simulink model "KUKA_EE_Controller_v22_orbital_verification2"  (R2024a)
settings: Solver=VariableStepAuto  StartTime=0.0  StopTime=120  FixedStep=0.01  RelTol=1e-3
InitFcn:
  | %rho_0t=[0.29;0.29;0.29]; %m
  | %V_0t=[-0.001;-0.001;0];%[-0.0005;-0.0005;0];
  | %w_t=[0;0;-0.002];
  | 
  | 
  | %rho_0t=[0.3;0.3;0.2]; %m
  | %V_0t=[-0.001;-0.001;0];%[-0.0005;-0.0005;0];
  | %w_t=[0;0;-0.001];
values from neighbouring files (symbols this model uses):
  e_orbit = 0    [Initiate_FQ.m]
  e_orbit_t = (mu_orbit_t^2/mu_earth)/radius_orbit_t-1    [Initiate_FQ.m]
  g_cm = zeros(4,4,n)    [Initiate_KUKA_inv.m]    (also in KUKA_Main.m)
  M0 = M_temp.M0.data(:,:,1)    [Initiate_FQ.m]    (also in KUKA_Main.m)
  m0 = robot.Bodies{1,n+1}.Mass    [Initiate_KUKA_inv.m]    (also in KUKA_Main.m)
  m0_frak = diag_M(1:6,1:6)    [Initiate_KUKA_inv.m]
  M0m = M_temp.M0m.data(:,:,1)    [Initiate_FQ.m]    (also in KUKA_Main.m)
  m_diag = diag_M(7:end,7:end)    [Initiate_KUKA_inv.m]
  Mean_Anomaly0 = MeanAnomaly(e_orbit,E0)    [Initiate_FQ.m]
  Mean_Anomaly0_t = MeanAnomaly(e_orbit,E0)    [Initiate_FQ.m]
  Mm = simplify(transpose(Xi_m)*transpose(Lm)*diagM*Lm*Xi_m)    [KUKA_Main.m]
  mm = zeros(1,n)    [Initiate_KUKA_inv.m]    (also in KUKA_Main.m)
  mu = P0    [Initiate_FQ.m]    (also in Initiate_KUKA_inv.m = zeros(6,1); KUKA_Main.m = P)
  mu_earth = 3.986004418*10^14    (= 398600441800000)    [Initiate_FQ.m]
  mu_orbit = sqrt(radius_orbit*mu_earth)    [Initiate_FQ.m]
  mu_orbit_t = radius_orbit_t*vel_orbit_t    [Initiate_FQ.m]
  n_orbit = (mu_earth^2)/(mu_orbit^3)    [Initiate_FQ.m]
  n_orbit_t = (mu_earth^2)/(mu_orbit^3)    [Initiate_FQ.m]
  q_dot_m = [0;0;0;0;0;0;0]    [Initiate_FQ.m]    (also in Initiate_KUKA_inv.m; KUKA_Main.m = [qdot1;qdot2;qdot3;qdot4;qdot5;qdot6;qdot7])
  q_m = [0.2;1.2;0.3;2.5;0.5;1.5;0.6]    [Initiate_FQ.m]    (also in Initiate_KUKA_inv.m = [0;0;0;0;0;0;0]; KUKA_Main.m = [q_m1;q_m2;q_m3;q_m4;q_m5;q_m6;q_m7])
  sc_size = 1    [Initiate_KUKA_inv.m]    (also in KUKA_Main.m)
  theta0 = 0    [Initiate_FQ.m]
  theta0_t = 0    [Initiate_FQ.m]
  V_I0 = [-0.0001;-0.0001;0.0;-0.001;0.001;0.002]    [Initiate_FQ.m]    (also in Initiate_KUKA_inv.m = [0;0;0;0;0;0]; KUKA_Main.m = [0;0;0;0;0;0])
  Xi_m = Xi_m(1:robot.n*6,1:robot.n)    [KUKA_Main.m]
  Xi_m_matrix = zeros(6*n,n)    [Initiate_KUKA_inv.m]    (also in KUKA_Main.m)
undefined symbols (not defined in the file or in its folder): g_cm0, I0, Im, X, Y, Z
libraries: nesl_utility x121, sm_lib x101, simulink x12, robotcorelib x7
(part 1 of 4)
settings Model: Creator=Bmmog  LastModifiedBy=Bmmog
settings SolverCC: ZeroCrossAlgorithm=Adaptive
settings DataIOCC: ReturnWorkspaceOutputsName=tp1ae71780_9f9b_41fc_80d6_93119145c185
settings DebuggingCC: UnconnectedInputMsg=warning  UnconnectedOutputMsg=warning  UnconnectedLineMsg=warning
settings ModelReferenceCC: EnableRefExpFcnMdlSchedulingChecks=on
settings RTWCC: GPUComputeCapability=3.5  DLArmComputeVersion=19.05
settings ExplorerConfigSet: InternalSimMechanicsExplorerSettings="<ExplorerConfiguration><canonicalview>default</canonicalview><AnimationSetting><BasePlaybackSpeed>1.0</BasePlaybackSpeed><PlaybackSpeedFactor>1.0</PlaybackSpeedFactor></AnimationSetting><TilePanel><TileInfo><Tiles Columns=\"1\" Count=\"1\" Rows=\"1\"><Column Weight=\"1\"/><Row Weight=\"1\"/><Tile Height=\"1\" Width=\"1\" X=\"0\" Y=\"0\"/></Tiles></TileInfo><SceneInfo><SceneViewer><BGColor><R>0.60000002384185791</R><G>0.60000002384185791</G><B>0.60000002384185791</B></BGColor><Camera><DoPerspective>on</DoPerspective><Position><X>-173.772038606457443</X><Y>1.13588376088164722</Y><Z>-1.92129485014535106</Z></Position><Center><X>-175.192222749432915</X><Y>4.39746342785919353</Y><Z>-3.56215931868599078</Z></Center><Up><X>0.0771327039681207333</X><Y>0.474680075340175867</Y><Z>0.876772132343182631</Z></Up><ViewLimDist>1</ViewLimDist><YLim>0.466307658154998583</YLim><XLim>0.468380136635687505</XLim></Camera></SceneViewer></SceneInfo></TilePanel><MechEditorPanel><Cameras><Camera><Id>Camera1</Id><Value><Name>Camera1</Name><NativeCamera><PositionTrackingFeature>Target.Target.Frame1</PositionTrackingFeature><CenterTrackingFeature/><UpVectorTrackingFeature/><CenterTrackingOrigin>on</CenterTrackingOrigin><UpVectorTrackingDirection>+X</UpVectorTrackingDirection></NativeCamera></Value></Camera></Cameras><GfxPanelCameraMap><MapElement CameraMLId=\"Camera1\" GfxPanelIndex=\"0\"/></GfxPanelCameraMap><VideoCreator><PlaybackSpeedRatio>1.0</PlaybackSpeedRatio><FrameRate>30</FrameRate><VideoFormat>Motion JPEG AVI</VideoFormat><FrameSize>auto</FrameSize></VideoCreator></MechEditorPanel></ExplorerConfiguration>"

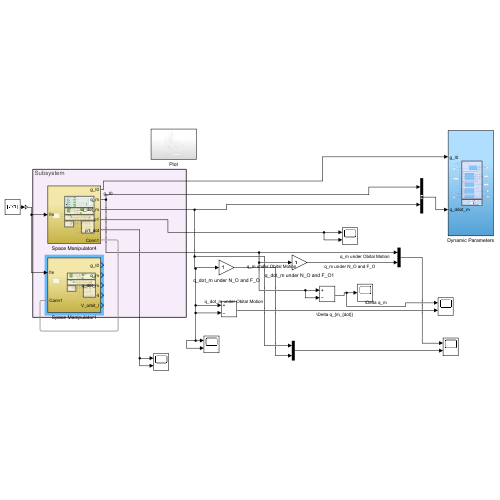
[thumbnail: Simulink's stored preview of the top-level diagram]
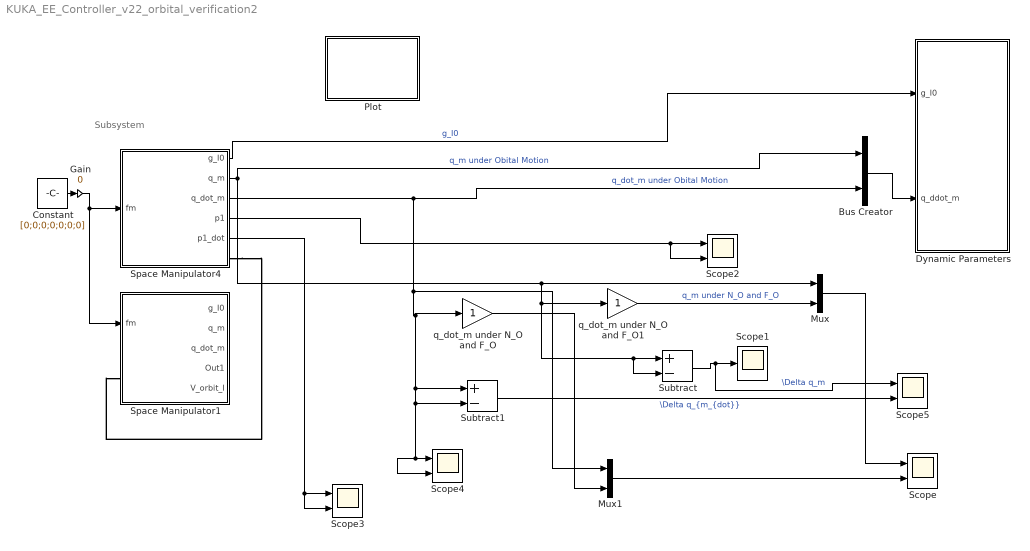
== system KUKA_EE_Controller_v22_orbital_verification2 ==
  note: Subsystem
  Bus Creator : BusCreator  Inputs=2
  Constant : Constant  Value=[0;0;0;0;0;0;0]
  Dynamic Parameters : Subsystem
  Gain : Gain  Gain=0
  Mux : Mux  Inputs=2
  Mux1 : Mux  Inputs=2
  Plot : Subsystem
  Scope{,2..5} (5 alike) : Scope  NumInputPorts=2
  Scope1 : Scope
  Space Manipulator1 : Subsystem
  Space Manipulator4 : Subsystem
  Subtract : Sum  Inputs=+-
  Subtract1 : Sum  Inputs=+-
  q_dot_m under N_O and F_O : Gain
  q_dot_m under N_O and F_O1 : Gain
  wires:
  Space Manipulator4/1(g_I0) -> Dynamic Parameters/1(g_I0)  "g_I0"
  Bus Creator/1 -> Dynamic Parameters/2(q_ddot_m)
  Gain/1 -> Space Manipulator1/1(fm), Space Manipulator4/1(fm)
  Space Manipulator4/2(q_m) -> Bus Creator/1, Mux/1, Subtract/2, Subtract/1, q_dot_m under N_O and F_O1/1  "q_m under Obital Motion"
  Space Manipulator4/3(q_dot_m) -> Bus Creator/2, q_dot_m under N_O and F_O/1, Subtract1/1, Scope4/2, Scope4/1, Subtract1/2, Mux1/1  "q_dot_m under Obital Motion"
  Constant/1 -> Gain/1
  Subtract/1 -> Scope5/1, Scope1/1  "\\Delta q_m"
  Space Manipulator4/4(p1) -> Scope2/2, Scope2/1
  Space Manipulator4/5(p1_dot) -> Scope3/2, Scope3/1
  Mux/1 -> Scope/1
  Mux1/1 -> Scope/2
  Subtract1/1 -> Scope5/2  "\\Delta q_{m_{dot}}"
  q_dot_m under N_O and F_O/1 -> Mux1/2
  q_dot_m under N_O and F_O1/1 -> Mux/2  "q_m under N_O and F_O"
  connections:
  Space Manipulator4/RConn1 -- Space Manipulator1/LConn1

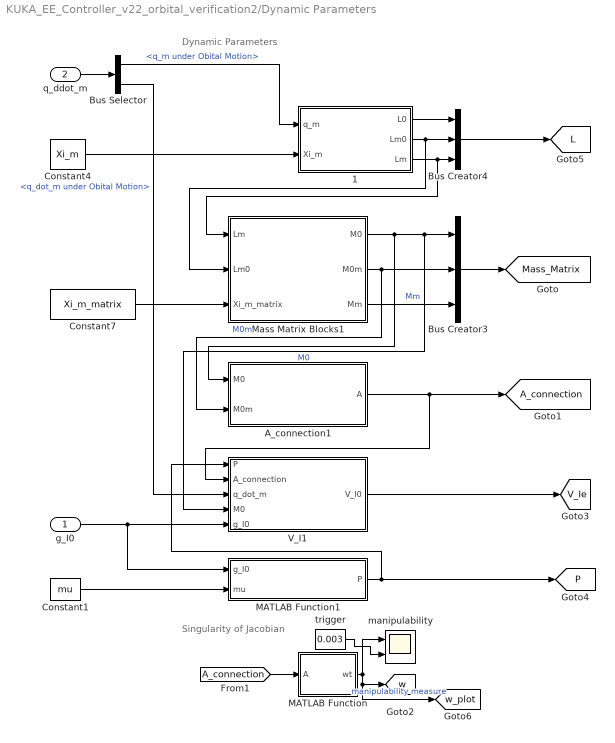
== system KUKA_EE_Controller_v22_orbital_verification2/Dynamic Parameters ==
  note: Singularity of Jacobian
  note: Dynamic Parameters
  g_I0 : Inport
  q_ddot_m : Inport  Port=2
  " 1" : MATLAB Function  TreatAsAtomicUnit=on
  A_connection1 : Subsystem
  Bus Creator3 : BusCreator  Inputs=M0,M0m,Mm
  Bus Creator4 : BusCreator  Inputs=3
  Bus Selector : BusSelector  OutputSignals=q_m under Obital Motion,q_dot_m under Obital Motion
  Constant1 : Constant  Value=mu
  Constant4 : Constant  Value=Xi_m
  Constant7 : Constant  Value=Xi_m_matrix
  MATLAB Function : MATLAB Function  TreatAsAtomicUnit=on
  MATLAB Function1 : MATLAB Function  TreatAsAtomicUnit=on
  Mass Matrix Blocks1 : Subsystem
  V_I1 : MATLAB Function  TreatAsAtomicUnit=on
  manipulability : Scope  NumInputPorts=2
  trigger : Constant  Value=0.003
  tag scope: A_connection=global, L=global, Mass_Matrix=global, P=global, V_Ie=global, w=global, w_plot=global
  wires:
  MATLAB Function1/1(P) -> V_I1/1(P), [P]
  Constant1/1 -> MATLAB Function1/2(mu)
  g_I0/1 -> MATLAB Function1/1(g_I0), V_I1/5(g_I0)
  A_connection1/1(A) -> [A_connection], V_I1/2(A_connection)
  Mass Matrix Blocks1/1(M0) -> A_connection1/1(M0), V_I1/4(M0), Bus Creator3/1  "M0"
  Mass Matrix Blocks1/3(Mm) -> Bus Creator3/3  "Mm"
  Bus Creator3/1 -> [Mass_Matrix]
  Bus Creator4/1 -> [L]
  q_ddot_m/1 -> Bus Selector/1
  " 1"/2(Lm0) -> Mass Matrix Blocks1/2(Lm0), Bus Creator4/2
  " 1"/1(L0) -> Bus Creator4/1
  Constant4/1 -> " 1"/2(Xi_m)
  " 1"/3(Lm) -> Bus Creator4/3, Mass Matrix Blocks1/1(Lm)
  Constant7/1 -> Mass Matrix Blocks1/3(Xi_m_matrix)
  Mass Matrix Blocks1/2(M0m) -> Bus Creator3/2, A_connection1/2(M0m)  "M0m"
  Bus Selector/2 -> V_I1/3(q_dot_m)  "<q_dot_m under Obital Motion>"
  Bus Selector/1 -> " 1"/1(q_m)  "<q_m under Obital Motion>"
  MATLAB Function/1(wt) -> [w_plot], [w], manipulability/1  "manipulability measure"
  [A_connection] -> MATLAB Function/1(A)
  trigger/1 -> manipulability/2
  V_I1/1(V_I0) -> [V_Ie]

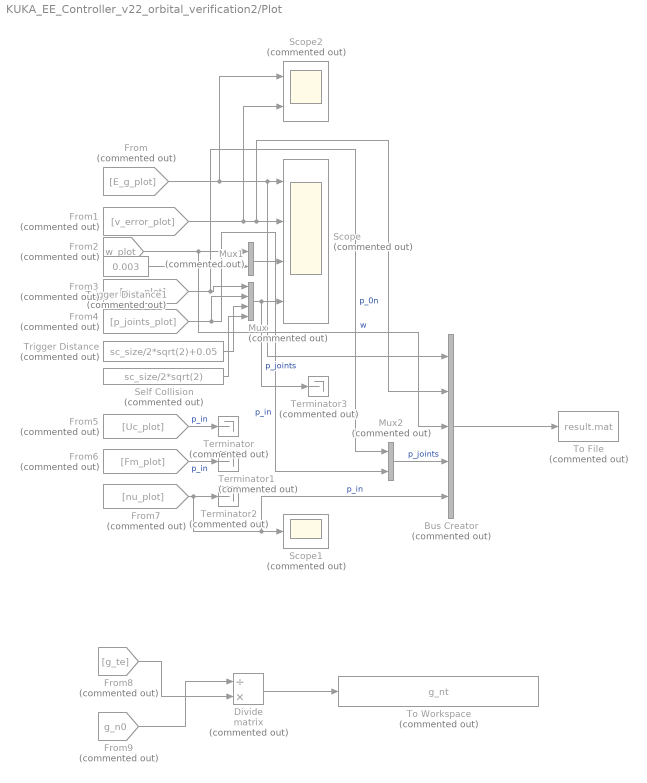
== system KUKA_EE_Controller_v22_orbital_verification2/Plot ==
  Bus Creator : BusCreator  Commented=on  Inputs=5
  Divide : Product  Commented=on  Inputs=/*  Multiplication=Matrix(*)
  From : From  Commented=on  GotoTag=E_g_plot
  From1 : From  Commented=on  GotoTag=v_error_plot
  From2 : From  Commented=on  GotoTag=w_plot  TagVisibility=global
  From3 : From  Commented=on  GotoTag=p_e_plot
  From4 : From  Commented=on  GotoTag=p_joints_plot
  From5 : From  Commented=on  GotoTag=Uc_plot
  From6 : From  Commented=on  GotoTag=Fm_plot
  From7 : From  Commented=on  GotoTag=nu_plot
  From8 : From  Commented=on  GotoTag=g_te
  From9 : From  Commented=on  GotoTag=g_n0  TagVisibility=global
  Mux : Mux  Commented=on  Inputs=[1 4 1 1]
  Mux1 : Mux  Commented=on  Inputs=2
  Mux2 : Mux  Commented=on  Inputs=2
  Scope : Scope  Commented=on  NumInputPorts=4
  Scope1 : Scope  Commented=on
  Scope2 : Scope  Commented=on  NumInputPorts=2
  Self Collision : Constant  Commented=on  Value=sc_size/2*sqrt(2)
  Terminator{,1..3} (4 alike) : Terminator  Commented=on
  To File : ToFile  Commented=on  Filename=result.mat
  To Workspace : ToWorkspace  Commented=on  VariableName=g_nt  SaveFormat=Timeseries  SampleTime=-1
  Trigger Distance : Constant  Commented=on  Value=sc_size/2*sqrt(2)+0.05
  Trigger Distance1 : Constant  Commented=on  Value=0.003
  wires:
  From/1 -> Scope2/1, Bus Creator/1, Scope/1
  From1/1 -> Scope2/2, Bus Creator/2, Scope/2
  From2/1 -> Bus Creator/3, Mux1/1  "w"
  From3/1 -> Mux2/1, Mux/1  "p_0n"
  From4/1 -> Mux/2, Mux2/2  "p_in"
  Mux/1 -> Scope/4, Terminator3/1  "p_joints"
  Trigger Distance/1 -> Mux/3
  From5/1 -> Terminator/1  "p_in"
  From6/1 -> Terminator1/1  "p_in"
  From7/1 -> Bus Creator/5, Scope1/1, Terminator2/1  "p_in"
  Self Collision/1 -> Mux/4
  Trigger Distance1/1 -> Mux1/2
  Mux1/1 -> Scope/3
  Bus Creator/1 -> To File/1
  Mux2/1 -> Bus Creator/4  "p_joints"
  From8/1 -> Divide/2
  From9/1 -> Divide/1
  Divide/1 -> To Workspace/1

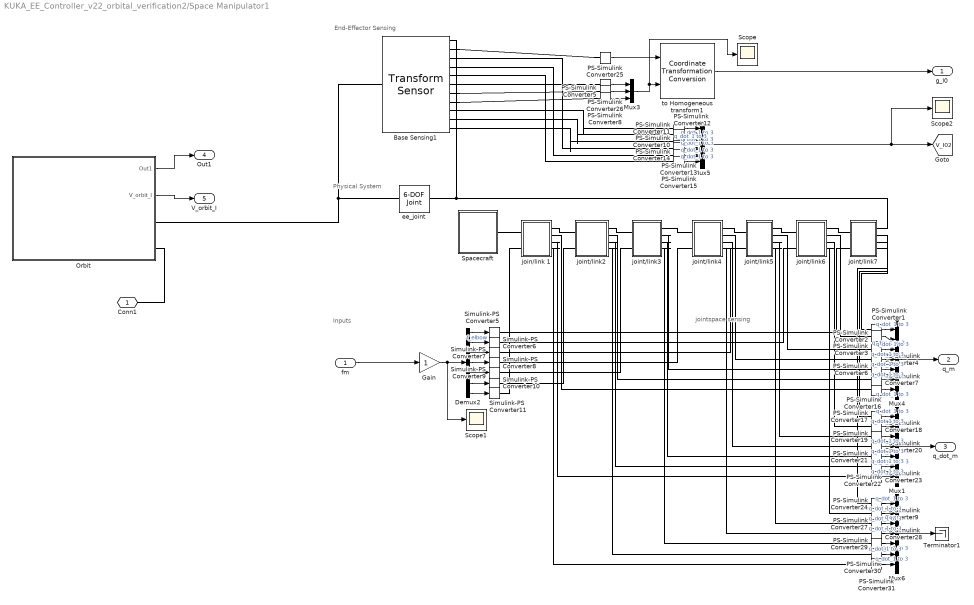
== system KUKA_EE_Controller_v22_orbital_verification2/Space Manipulator1 ==
  note: End-Effector Sensing
  note: Inputs
  note: jointspace sensing
  note: Physical System
  fm : Inport
  Base Sensing1 : sm_lib/Frames and Transforms/Transform Sensor  MeasurementFrame=NonRotatingBase  RotationSequence=XYZ  SenseAngle=off  SenseAxis=off  SenseQ=off  SenseR=on  SenseRotationSequence=off  SenseOmegaX=on  SenseOmegaY=on  SenseOmegaZ=on  SenseOmega=off  SenseQDot=off  SenseRDot=off  SenseRotationSequenceDot=off  SenseAlphaX=off  SenseAlphaY=off  SenseAlphaZ=off  SenseAlpha=off  SenseQDDot=off  SenseRDDot=off  SenseX=on  SenseY=on  SenseZ=on  SenseXYZ=off  SenseRad=off  SenseAzim=off  SenseDist=off  SenseInc=off  SenseXDot=on  SenseYDot=on  SenseZDot=on  SenseXYZDot=off  SenseRadDot=off  SenseAzimDot=off  SenseDistDot=off  SenseIncDot=off  SenseXDDot=off  SenseYDDot=off  SenseZDDot=off  SenseXYZDDot=off  SenseRadDDot=off  SenseAzimDDot=off  SenseDistDDot=off  SenseIncDDot=off
  Demux2 : Demux  Outputs=7
  Gain : Gain
  Mux1 : Mux  Inputs=7
  Mux3 : Mux  Inputs=3
  Mux4 : Mux  Inputs=7
  Mux5 : Mux  Inputs=6
  Mux6 : Mux  Inputs=7
  Orbit : Subsystem
  PS-Simulink Converter{1..31} (31 alike) : nesl_utility/PS-Simulink Converter  PhysicalDomain=network_engine_domain  SubClassName=ps_output  LeftPortType=input  RightPortType=output  PseudoPeriodic=off  Frequencies=[]  VectorFormat=1-D array  Unit=inherit  AffineConversion=off
  Scope : Scope
  Scope1 : Scope
  Scope2 : Scope
  Simulink-PS Converter{5..11} (7 alike) : nesl_utility/Simulink-PS Converter  PhysicalDomain=network_engine_domain  SubClassName=ps_input  LeftPortType=input  RightPortType=output  PseudoPeriodic=off  Frequencies=[]  NoiseDistribution=none  NoiseParameters=[]  Unit=1  AffineConversion=off  FilteringAndDerivatives=provide  SimscapeFilterOrder=1  InputFilterTimeConstant=0.001  UdotUserProvided=0
  Spacecraft : Subsystem
  Terminator1 : Terminator
  ee_joint : sm_lib/Joints/6-DOF Joint  JointMode=Normal  CompositeWrenchDir=FollowerOnBase  CompositeWrenchFrame=BaseFrame  SenseConstraintForce=off  SenseConstraintTorque=off  SenseTotalForce=off  SenseTotalTorque=off  PxPositionTargetSpecify=on  PxPositionTargetPriority=High  PxPositionTargetValue=0  PxPositionTargetValueUnits=m  PxVelocityTargetSpecify=on  PxVelocityTargetPriority=High  PxVelocityTargetValue=V_I0(1)  PxVelocityTargetValueUnits=m/s  PxEquilibriumPosition=0  PxEquilibriumPositionUnits=m  PxSpringStiffness=0  PxSpringStiffnessUnits=N/m  PxDampingCoefficient=0  PxDampingCoefficientUnits=N/(m/s)  PxLowerLimitSpecify=off  PxLowerLimitBound=-1  PxLowerLimitBoundUnits=m  PxLowerLimitStiffness=1e6  PxLowerLimitStiffnessUnits=N/m  PxLowerLimitDamping=1e3  PxLowerLimitDampingUnits=N/(m/s)  PxLowerLimitTransitionRegionWidth=1e-4  PxLowerLimitTransitionRegionWidthUnits=m  PxUpperLimitSpecify=off  PxUpperLimitBound=1  PxUpperLimitBoundUnits=m  PxUpperLimitStiffness=1e6  PxUpperLimitStiffnessUnits=N/m  PxUpperLimitDamping=1e3  PxUpperLimitDampingUnits=N/(m/s)  PxUpperLimitTransitionRegionWidth=1e-4  PxUpperLimitTransitionRegionWidthUnits=m  PxTorqueActuationMode=ComputedTorque  PxMotionActuationMode=ComputedMotion  PxSensePosition=off  PxSenseVelocity=off  PxSenseAcceleration=off  PxSenseTorqueForce=off  PxSenseLowerLimitTorqueForce=off  PxSenseUpperLimitTorqueForce=off  PyPositionTargetSpecify=on  PyPositionTargetPriority=High  PyPositionTargetValue=0  PyPositionTargetValueUnits=m  PyVelocityTargetSpecify=on  PyVelocityTargetPriority=High  PyVelocityTargetValue=V_I0(2)  PyVelocityTargetValueUnits=m/s  PyEquilibriumPosition=0  PyEquilibriumPositionUnits=m  PySpringStiffness=0  PySpringStiffnessUnits=N/m  PyDampingCoefficient=0  PyDampingCoefficientUnits=N/(m/s)  PyLowerLimitSpecify=off  PyLowerLimitBound=-1  PyLowerLimitBoundUnits=m  PyLowerLimitStiffness=1e6  PyLowerLimitStiffnessUnits=N/m  PyLowerLimitDamping=1e3  PyLowerLimitDampingUnits=N/(m/s)  PyLowerLimitTransitionRegionWidth=1e-4  PyLowerLimitTransitionRegionWidthUnits=m  PyUpperLimitSpecify=off  PyUpperLimitBound=1  PyUpperLimitBoundUnits=m  PyUpperLimitStiffness=1e6  PyUpperLimitStiffnessUnits=N/m  PyUpperLimitDamping=1e3  PyUpperLimitDampingUnits=N/(m/s)  PyUpperLimitTransitionRegionWidth=1e-4  PyUpperLimitTransitionRegionWidthUnits=m  PyTorqueActuationMode=ComputedTorque  PyMotionActuationMode=ComputedMotion  PySensePosition=off  PySenseVelocity=off  PySenseAcceleration=off  PySenseTorqueForce=off  PySenseLowerLimitTorqueForce=off  PySenseUpperLimitTorqueForce=off  PzPositionTargetSpecify=on  PzPositionTargetPriority=High  PzPositionTargetValue=0  PzPositionTargetValueUnits=m  PzVelocityTargetSpecify=on  PzVelocityTargetPriority=High  PzVelocityTargetValue=V_I0(3)  PzVelocityTargetValueUnits=m/s  PzEquilibriumPosition=0  PzEquilibriumPositionUnits=m  PzSpringStiffness=0  PzSpringStiffnessUnits=N/m  PzDampingCoefficient=0  PzDampingCoefficientUnits=N/(m/s)  PzLowerLimitSpecify=off  PzLowerLimitBound=-1  PzLowerLimitBoundUnits=m  PzLowerLimitStiffness=1e6  PzLowerLimitStiffnessUnits=N/m  PzLowerLimitDamping=1e3  PzLowerLimitDampingUnits=N/(m/s)  PzLowerLimitTransitionRegionWidth=1e-4  PzLowerLimitTransitionRegionWidthUnits=m  PzUpperLimitSpecify=off  PzUpperLimitBound=1  PzUpperLimitBoundUnits=m  PzUpperLimitStiffness=1e6  PzUpperLimitStiffnessUnits=N/m  PzUpperLimitDamping=1e3  PzUpperLimitDampingUnits=N/(m/s)  PzUpperLimitTransitionRegionWidth=1e-4  PzUpperLimitTransitionRegionWidthUnits=m  PzTorqueActuationMode=ComputedTorque  PzMotionActuationMode=ComputedMotion  PzSensePosition=off  PzSenseVelocity=off  PzSenseAcceleration=off  PzSenseTorqueForce=off  PzSenseLowerLimitTorqueForce=off  PzSenseUpperLimitTorqueForce=off  SphPositionTargetSpecify=on  SphPositionTargetPriority=High  SphPositionTargetRotationMethod=RotationSequence  SphPositionTargetFollAlignAxisA=+X  SphPositionTargetBaseAlignAxisA=+Y  SphPositionTargetFollAlignAxisB=+Y  SphPositionTargetBaseAlignAxisB=+Z  SphPositionTargetRotationStandardAxis=+Z  SphPositionTargetRotationAngle=0.0  SphPositionTargetRotationAngleUnits=deg  SphPositionTargetRotationArbitraryAxis=[0 0 1]  SphPositionTargetRotationSequenceAxes=FollowerAxes  SphPositionTargetRotationSequence=ZYX  SphPositionTargetRotationSequenceAngles=[0 0 0]  SphPositionTargetRotationSequenceAnglesUnits=rad  SphPositionTargetRotationMatrix=[1 0 0; 0 1 0; 0 0 1]  SphPositionTargetQuaternion=[1 0 0 0]  SphVelocityTargetSpecify=on  SphVelocityTargetPriority=High  SphVelocityTargetValue=[V_I0(4) V_I0(5) V_I0(6)]  SphVelocityTargetValueUnits=rad/s  SphVelocityTargetInFollowerFrame=on  SphEqPosRotationMethod=None  SphEqPosFollAlignAxisA=+X  SphEqPosBaseAlignAxisA=+Y  SphEqPosFollAlignAxisB=+Y  SphEqPosBaseAlignAxisB=+Z  SphEqPosRotationStandardAxis=+Z  SphEqPosRotationAngle=0.0  SphEqPosRotationAngleUnits=deg  SphEqPosRotationArbitraryAxis=[0 0 1]  SphEqPosRotationSequenceAxes=FollowerAxes  SphEqPosRotationSequence=XYX  SphEqPosRotationSequenceAngles=[0 0 0]  SphEqPosRotationSequenceAnglesUnits=deg  SphEqPosRotationMatrix=[1 0 0; 0 1 0; 0 0 1]  SphEqPosQuaternion=[1 0 0 0]  SphSpringStiffness=0  SphSpringStiffnessUnits=N*m/deg  SphDampingCoefficient=0  SphDampingCoefficientUnits=N*m/(deg/s)  SphLowerLimitSpecify=off  SphLowerLimitBound=15  SphLowerLimitBoundUnits=deg  SphLowerLimitStiffness=1e4  SphLowerLimitStiffnessUnits=N*m/deg  SphLowerLimitDamping=10  SphLowerLimitDampingUnits=N*m/(deg/s)  SphLowerLimitTransitionRegionWidth=0.1  SphLowerLimitTransitionRegionWidthUnits=deg  SphUpperLimitSpecify=off  SphUpperLimitBound=45  SphUpperLimitBoundUnits=deg  SphUpperLimitStiffness=1e4  SphUpperLimitStiffnessUnits=N*m/deg  SphUpperLimitDamping=10  SphUpperLimitDampingUnits=N*m/(deg/s)  SphUpperLimitTransitionRegionWidth=0.1  SphUpperLimitTransitionRegionWidthUnits=deg  SphTorqueActuationMode=NoTorque  SphActuateTorqueX=off  SphActuateTorqueY=off  SphActuateTorqueZ=off  SphActuateTorque=off  SphActuationFrame=BaseFrame  SphSensePosition=off  SphSenseVelocityX=off  SphSenseVelocityY=off  SphSenseVelocityZ=off  SphSenseVelocity=off  SphSenseAccelerationX=off  SphSenseAccelerationY=off  SphSenseAccelerationZ=off  SphSenseAcceleration=off  SphSenseLowerLimitTorqueMag=off  SphSenseUpperLimitTorqueMag=off  SphSensingFrame=BaseFrame
  join/link 1 : Subsystem
  joint/link2 : Subsystem
  joint/link3 : Subsystem
  joint/link4 : Subsystem
  joint/link5 : Subsystem
  joint/link6 : Subsystem
  joint/link7 : Subsystem
  to Homogeneous transform1 : robotcorelib/Coordinate Transformation Conversion  InputRepresentation=Rotation Matrix  InputEulerSequence=ZYX  ShowTrVecInputPort=on  OutputRepresentation=Homogeneous Transformation  OutputEulerSequence=ZYX  ShowTrVecOutputPort=on  SimulateUsing=Code generation
  Conn1 : PMIOPort  Side=Left
  g_I0 : Outport
  q_m : Outport  Port=2
  q_dot_m : Outport  Port=3
  Out1 : Outport  Port=4
  V_orbit_I : Outport  Port=5
  tag scope: V_I02=global
  wires:
  Mux5/1 -> Scope2/1, [V_I02]
  PS-Simulink Converter19/1 -> Mux1/3  "q_dot_1 to 3"
  PS-Simulink Converter17/1 -> Mux1/1  "q_dot_1 to 3"
  PS-Simulink Converter22/1 -> Mux1/6  "q_dot_1 to 3"
  PS-Simulink Converter29/1 -> Mux6/5  "q_dot_1 to 3"
  PS-Simulink Converter20/1 -> Mux1/4  "q_dot_1 to 3"
  Mux6/1 -> Terminator1/1
  PS-Simulink Converter24/1 -> Mux6/1  "q_dot_1 to 3"
  Mux1/1 -> q_dot_m/1
  Mux4/1 -> q_m/1
  PS-Simulink Converter28/1 -> Mux6/4  "q_dot_1 to 3"
  PS-Simulink Converter16/1 -> Mux4/7  "q_dot_1 to 3"
  PS-Simulink Converter23/1 -> Mux1/7  "q_dot_1 to 3"
  PS-Simulink Converter21/1 -> Mux1/5  "q_dot_1 to 3"
  PS-Simulink Converter4/1 -> Mux4/4  "q_dot_1 to 3"
  PS-Simulink Converter2/1 -> Mux4/2  "q_dot_1 to 3"
  PS-Simulink Converter7/1 -> Mux4/6  "q_dot_1 to 3"
  PS-Simulink Converter9/1 -> Mux6/2  "q_dot_1 to 3"
  PS-Simulink Converter31/1 -> Mux6/7  "q_dot_1 to 3"
  PS-Simulink Converter18/1 -> Mux1/2  "q_dot_1 to 3"
  PS-Simulink Converter3/1 -> Mux4/3  "q_dot_1 to 3"
  PS-Simulink Converter30/1 -> Mux6/6  "q_dot_1 to 3"
  PS-Simulink Converter6/1 -> Mux4/5  "q_dot_1 to 3"
  PS-Simulink Converter1/1 -> Mux4/1  "q_dot_1 to 3"
  PS-Simulink Converter27/1 -> Mux6/3  "q_dot_1 to 3"
  Demux2/5 -> Simulink-PS Converter9/1
  Demux2/2 -> Simulink-PS Converter6/1  "f_elbow"
  Demux2/6 -> Simulink-PS Converter10/1
  PS-Simulink Converter5/1 -> Mux3/2
  PS-Simulink Converter11/1 -> Mux5/1  "q_dot_1 to 3"
  Demux2/4 -> Simulink-PS Converter8/1
  PS-Simulink Converter14/1 -> Mux5/5  "q_dot_1 to 3"
  Demux2/7 -> Simulink-PS Converter11/1
  PS-Simulink Converter26/1 -> Mux3/1
  PS-Simulink Converter13/1 -> Mux5/4  "q_dot_1 to 3"
  to Homogeneous transform1/1 -> g_I0/1
  PS-Simulink Converter12/1 -> Mux5/2  "q_dot_1 to 3"
  Mux3/1 -> to Homogeneous transform1/2, Scope/1
  PS-Simulink Converter8/1 -> Mux3/3
  Gain/1 -> Demux2/1, Scope1/1
  PS-Simulink Converter25/1 -> to Homogeneous transform1/1
  fm/1 -> Gain/1
  PS-Simulink Converter10/1 -> Mux5/3  "q_dot_1 to 3"
  PS-Simulink Converter15/1 -> Mux5/6  "q_dot_1 to 3"
  Demux2/3 -> Simulink-PS Converter7/1
  Demux2/1 -> Simulink-PS Converter5/1
  Orbit/1(Out1) -> Out1/1
  Orbit/2(V_orbit_I) -> V_orbit_I/1
  connections:
  join/link 1/RConn3 -- PS-Simulink Converter23/LConn1
  joint/link2/RConn3 -- PS-Simulink Converter22/LConn1
  join/link 1/RConn4 -- PS-Simulink Converter31/LConn1
  joint/link2/RConn4 -- PS-Simulink Converter30/LConn1
  PS-Simulink Converter7/LConn1 -- joint/link2/RConn2
  join/link 1/RConn2 -- PS-Simulink Converter16/LConn1
  joint/link3/LConn1 -- joint/link2/RConn1
  Simulink-PS Converter10/RConn1 -- joint/link2/LConn2
  join/link 1/RConn1 -- joint/link2/LConn1
  join/link 1/LConn1 -- Spacecraft/RConn1
  join/link 1/LConn2 -- Simulink-PS Converter11/RConn1
  joint/link7/RConn4 -- PS-Simulink Converter24/LConn1
  joint/link7/RConn3 -- PS-Simulink Converter17/LConn1
  joint/link7/RConn2 -- PS-Simulink Converter1/LConn1
  joint/link6/LConn2 -- Simulink-PS Converter6/RConn1
  joint/link6/RConn2 -- PS-Simulink Converter2/LConn1
  joint/link6/RConn1 -- joint/link7/LConn1
  joint/link3/RConn4 -- PS-Simulink Converter29/LConn1
  joint/link3/RConn3 -- PS-Simulink Converter21/LConn1
  joint/link3/RConn2 -- PS-Simulink Converter6/LConn1
  joint/link4/RConn4 -- PS-Simulink Converter28/LConn1
  joint/link4/RConn3 -- PS-Simulink Converter20/LConn1
  joint/link4/RConn2 -- PS-Simulink Converter4/LConn1
  joint/link5/RConn4 -- PS-Simulink Converter27/LConn1
  joint/link5/RConn3 -- PS-Simulink Converter19/LConn1
  joint/link5/RConn2 -- PS-Simulink Converter3/LConn1
  joint/link6/RConn4 -- PS-Simulink Converter9/LConn1
  joint/link6/RConn3 -- PS-Simulink Converter18/LConn1
  Simulink-PS Converter7/RConn1 -- joint/link5/LConn2
  Base Sensing1/RConn6 -- PS-Simulink Converter26/LConn1
  Base Sensing1/RConn8 -- PS-Simulink Converter8/LConn1
  Base Sensing1/RConn9 -- PS-Simulink Converter11/LConn1
  Base Sensing1/RConn4 -- PS-Simulink Converter14/LConn1
  Simulink-PS Converter5/RConn1 -- joint/link7/LConn2
  Base Sensing1/RConn3 -- PS-Simulink Converter13/LConn1
  Base Sensing1/RConn11 -- PS-Simulink Converter10/LConn1
  joint/link6/LConn1 -- joint/link5/RConn1
  Base Sensing1/RConn7 -- PS-Simulink Converter5/LConn1
  Base Sensing1/RConn5 -- PS-Simulink Converter15/LConn1
  joint/link5/LConn1 -- joint/link4/RConn1
  Base Sensing1/RConn2 -- PS-Simulink Converter25/LConn1
  Simulink-PS Converter8/RConn1 -- joint/link4/LConn2
  Simulink-PS Converter9/RConn1 -- joint/link3/LConn2
  Base Sensing1/RConn10 -- PS-Simulink Converter12/LConn1
  joint/link4/LConn1 -- joint/link3/RConn1
  joint/link7/RConn1 -- Base Sensing1/RConn1 -- ee_joint/RConn1
  Base Sensing1/LConn1 -- Orbit/RConn1 -- ee_joint/LConn1
  Conn1/RConn1 -- Orbit/RConn2

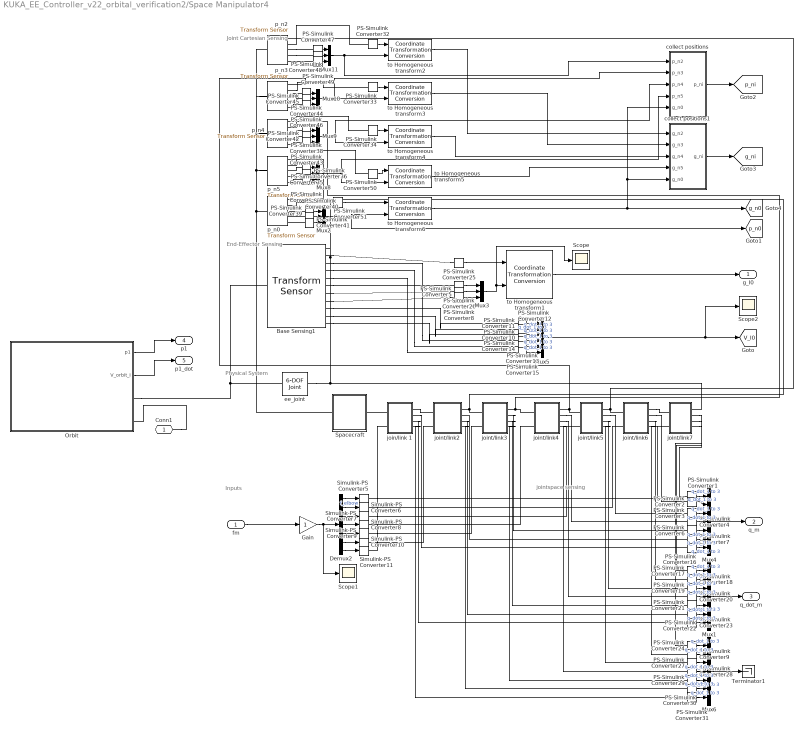
== system KUKA_EE_Controller_v22_orbital_verification2/Space Manipulator4 ==
  note: Physical System
  note: jointspace sensing
  note: Inputs
  note: End-Effector Sensing
  note: Joint Cartesian Sensing
  fm : Inport
  Base Sensing1 : sm_lib/Frames and Transforms/Transform Sensor  MeasurementFrame=NonRotatingBase  RotationSequence=XYZ  SenseAngle=off  SenseAxis=off  SenseQ=off  SenseR=on  SenseRotationSequence=off  SenseOmegaX=on  SenseOmegaY=on  SenseOmegaZ=on  SenseOmega=off  SenseQDot=off  SenseRDot=off  SenseRotationSequenceDot=off  SenseAlphaX=off  SenseAlphaY=off  SenseAlphaZ=off  SenseAlpha=off  SenseQDDot=off  SenseRDDot=off  SenseX=on  SenseY=on  SenseZ=on  SenseXYZ=off  SenseRad=off  SenseAzim=off  SenseDist=off  SenseInc=off  SenseXDot=on  SenseYDot=on  SenseZDot=on  SenseXYZDot=off  SenseRadDot=off  SenseAzimDot=off  SenseDistDot=off  SenseIncDot=off  SenseXDDot=off  SenseYDDot=off  SenseZDDot=off  SenseXYZDDot=off  SenseRadDDot=off  SenseAzimDDot=off  SenseDistDDot=off  SenseIncDDot=off
  Demux2 : Demux  Outputs=7
  Gain : Gain
  Mux1 : Mux  Inputs=7
  Mux{2..3,8..11} (6 alike) : Mux  Inputs=3
  Mux4 : Mux  Inputs=7
  Mux5 : Mux  Inputs=6
  Mux6 : Mux  Inputs=7
  Orbit : Subsystem
  PS-Simulink Converter{1..51} (51 alike) : nesl_utility/PS-Simulink Converter  PhysicalDomain=network_engine_domain  SubClassName=ps_output  LeftPortType=input  RightPortType=output  PseudoPeriodic=off  Frequencies=[]  VectorFormat=1-D array  Unit=inherit  AffineConversion=off
  Scope : Scope
  Scope1 : Scope
  Scope2 : Scope
  Simulink-PS Converter{5..11} (7 alike) : nesl_utility/Simulink-PS Converter  PhysicalDomain=network_engine_domain  SubClassName=ps_input  LeftPortType=input  RightPortType=output  PseudoPeriodic=off  Frequencies=[]  NoiseDistribution=none  NoiseParameters=[]  Unit=1  AffineConversion=off  FilteringAndDerivatives=provide  SimscapeFilterOrder=1  InputFilterTimeConstant=0.001  UdotUserProvided=0
  Spacecraft : Subsystem
  Terminator1 : Terminator
  collect positions : MATLAB Function  TreatAsAtomicUnit=on
  collect positions1 : MATLAB Function  TreatAsAtomicUnit=on
  ee_joint : sm_lib/Joints/6-DOF Joint  JointMode=Normal  CompositeWrenchDir=FollowerOnBase  CompositeWrenchFrame=BaseFrame  SenseConstraintForce=off  SenseConstraintTorque=off  SenseTotalForce=off  SenseTotalTorque=off  PxPositionTargetSpecify=on  PxPositionTargetPriority=High  PxPositionTargetValue=0  PxPositionTargetValueUnits=m  PxVelocityTargetSpecify=on  PxVelocityTargetPriority=High  PxVelocityTargetValue=V_I0(1)  PxVelocityTargetValueUnits=m/s  PxEquilibriumPosition=0  PxEquilibriumPositionUnits=m  PxSpringStiffness=0  PxSpringStiffnessUnits=N/m  PxDampingCoefficient=0  PxDampingCoefficientUnits=N/(m/s)  PxLowerLimitSpecify=off  PxLowerLimitBound=-1  PxLowerLimitBoundUnits=m  PxLowerLimitStiffness=1e6  PxLowerLimitStiffnessUnits=N/m  PxLowerLimitDamping=1e3  PxLowerLimitDampingUnits=N/(m/s)  PxLowerLimitTransitionRegionWidth=1e-4  PxLowerLimitTransitionRegionWidthUnits=m  PxUpperLimitSpecify=off  PxUpperLimitBound=1  PxUpperLimitBoundUnits=m  PxUpperLimitStiffness=1e6  PxUpperLimitStiffnessUnits=N/m  PxUpperLimitDamping=1e3  PxUpperLimitDampingUnits=N/(m/s)  PxUpperLimitTransitionRegionWidth=1e-4  PxUpperLimitTransitionRegionWidthUnits=m  PxTorqueActuationMode=ComputedTorque  PxMotionActuationMode=ComputedMotion  PxSensePosition=off  PxSenseVelocity=off  PxSenseAcceleration=off  PxSenseTorqueForce=off  PxSenseLowerLimitTorqueForce=off  PxSenseUpperLimitTorqueForce=off  PyPositionTargetSpecify=on  PyPositionTargetPriority=High  PyPositionTargetValue=0  PyPositionTargetValueUnits=m  PyVelocityTargetSpecify=on  PyVelocityTargetPriority=High  PyVelocityTargetValue=V_I0(2)  PyVelocityTargetValueUnits=m/s  PyEquilibriumPosition=0  PyEquilibriumPositionUnits=m  PySpringStiffness=0  PySpringStiffnessUnits=N/m  PyDampingCoefficient=0  PyDampingCoefficientUnits=N/(m/s)  PyLowerLimitSpecify=off  PyLowerLimitBound=-1  PyLowerLimitBoundUnits=m  PyLowerLimitStiffness=1e6  PyLowerLimitStiffnessUnits=N/m  PyLowerLimitDamping=1e3  PyLowerLimitDampingUnits=N/(m/s)  PyLowerLimitTransitionRegionWidth=1e-4  PyLowerLimitTransitionRegionWidthUnits=m  PyUpperLimitSpecify=off  PyUpperLimitBound=1  PyUpperLimitBoundUnits=m  PyUpperLimitStiffness=1e6  PyUpperLimitStiffnessUnits=N/m  PyUpperLimitDamping=1e3  PyUpperLimitDampingUnits=N/(m/s)  PyUpperLimitTransitionRegionWidth=1e-4  PyUpperLimitTransitionRegionWidthUnits=m  PyTorqueActuationMode=ComputedTorque  PyMotionActuationMode=ComputedMotion  PySensePosition=off  PySenseVelocity=off  PySenseAcceleration=off  PySenseTorqueForce=off  PySenseLowerLimitTorqueForce=off  PySenseUpperLimitTorqueForce=off  PzPositionTargetSpecify=on  PzPositionTargetPriority=High  PzPositionTargetValue=0  PzPositionTargetValueUnits=m  PzVelocityTargetSpecify=on  PzVelocityTargetPriority=High  PzVelocityTargetValue=V_I0(3)  PzVelocityTargetValueUnits=m/s  PzEquilibriumPosition=0  PzEquilibriumPositionUnits=m  PzSpringStiffness=0  PzSpringStiffnessUnits=N/m  PzDampingCoefficient=0  PzDampingCoefficientUnits=N/(m/s)  PzLowerLimitSpecify=off  PzLowerLimitBound=-1  PzLowerLimitBoundUnits=m  PzLowerLimitStiffness=1e6  PzLowerLimitStiffnessUnits=N/m  PzLowerLimitDamping=1e3  PzLowerLimitDampingUnits=N/(m/s)  PzLowerLimitTransitionRegionWidth=1e-4  PzLowerLimitTransitionRegionWidthUnits=m  PzUpperLimitSpecify=off  PzUpperLimitBound=1  PzUpperLimitBoundUnits=m  PzUpperLimitStiffness=1e6  PzUpperLimitStiffnessUnits=N/m  PzUpperLimitDamping=1e3  PzUpperLimitDampingUnits=N/(m/s)  PzUpperLimitTransitionRegionWidth=1e-4  PzUpperLimitTransitionRegionWidthUnits=m  PzTorqueActuationMode=ComputedTorque  PzMotionActuationMode=ComputedMotion  PzSensePosition=off  PzSenseVelocity=off  PzSenseAcceleration=off  PzSenseTorqueForce=off  PzSenseLowerLimitTorqueForce=off  PzSenseUpperLimitTorqueForce=off  SphPositionTargetSpecify=on  SphPositionTargetPriority=High  SphPositionTargetRotationMethod=RotationSequence  SphPositionTargetFollAlignAxisA=+X  SphPositionTargetBaseAlignAxisA=+Y  SphPositionTargetFollAlignAxisB=+Y  SphPositionTargetBaseAlignAxisB=+Z  SphPositionTargetRotationStandardAxis=+Z  SphPositionTargetRotationAngle=0.0  SphPositionTargetRotationAngleUnits=deg  SphPositionTargetRotationArbitraryAxis=[0 0 1]  SphPositionTargetRotationSequenceAxes=FollowerAxes  SphPositionTargetRotationSequence=ZYX  SphPositionTargetRotationSequenceAngles=[0 0 0]  SphPositionTargetRotationSequenceAnglesUnits=rad  SphPositionTargetRotationMatrix=[1 0 0; 0 1 0; 0 0 1]  SphPositionTargetQuaternion=[1 0 0 0]  SphVelocityTargetSpecify=on  SphVelocityTargetPriority=High  SphVelocityTargetValue=[V_I0(4) V_I0(5) V_I0(6)]  SphVelocityTargetValueUnits=rad/s  SphVelocityTargetInFollowerFrame=on  SphEqPosRotationMethod=None  SphEqPosFollAlignAxisA=+X  SphEqPosBaseAlignAxisA=+Y  SphEqPosFollAlignAxisB=+Y  SphEqPosBaseAlignAxisB=+Z  SphEqPosRotationStandardAxis=+Z  SphEqPosRotationAngle=0.0  SphEqPosRotationAngleUnits=deg  SphEqPosRotationArbitraryAxis=[0 0 1]  SphEqPosRotationSequenceAxes=FollowerAxes  SphEqPosRotationSequence=XYX  SphEqPosRotationSequenceAngles=[0 0 0]  SphEqPosRotationSequenceAnglesUnits=deg  SphEqPosRotationMatrix=[1 0 0; 0 1 0; 0 0 1]  SphEqPosQuaternion=[1 0 0 0]  SphSpringStiffness=0  SphSpringStiffnessUnits=N*m/deg  SphDampingCoefficient=0  SphDampingCoefficientUnits=N*m/(deg/s)  SphLowerLimitSpecify=off  SphLowerLimitBound=15  SphLowerLimitBoundUnits=deg  SphLowerLimitStiffness=1e4  SphLowerLimitStiffnessUnits=N*m/deg  SphLowerLimitDamping=10  SphLowerLimitDampingUnits=N*m/(deg/s)  SphLowerLimitTransitionRegionWidth=0.1  SphLowerLimitTransitionRegionWidthUnits=deg  SphUpperLimitSpecify=off  SphUpperLimitBound=45  SphUpperLimitBoundUnits=deg  SphUpperLimitStiffness=1e4  SphUpperLimitStiffnessUnits=N*m/deg  SphUpperLimitDamping=10  SphUpperLimitDampingUnits=N*m/(deg/s)  SphUpperLimitTransitionRegionWidth=0.1  SphUpperLimitTransitionRegionWidthUnits=deg  SphTorqueActuationMode=NoTorque  SphActuateTorqueX=off  SphActuateTorqueY=off  SphActuateTorqueZ=off  SphActuateTorque=off  SphActuationFrame=BaseFrame  SphSensePosition=off  SphSenseVelocityX=off  SphSenseVelocityY=off  SphSenseVelocityZ=off  SphSenseVelocity=off  SphSenseAccelerationX=off  SphSenseAccelerationY=off  SphSenseAccelerationZ=off  SphSenseAcceleration=off  SphSenseLowerLimitTorqueMag=off  SphSenseUpperLimitTorqueMag=off  SphSensingFrame=BaseFrame
  join/link 1 : Subsystem
  joint/link2 : Subsystem
  joint/link3 : Subsystem
  joint/link4 : Subsystem
  joint/link5 : Subsystem
  joint/link6 : Subsystem
  joint/link7 : Subsystem
  p_n{0,2..5} (5 alike) : sm_lib/Frames and Transforms/Transform Sensor  MeasurementFrame=Base  RotationSequence=XYZ  SenseAngle=off  SenseAxis=off  SenseQ=off  SenseR=on  SenseRotationSequence=off  SenseOmegaX=off  SenseOmegaY=off  SenseOmegaZ=off  SenseOmega=off  SenseQDot=off  SenseRDot=off  SenseRotationSequenceDot=off  SenseAlphaX=off  SenseAlphaY=off  SenseAlphaZ=off  SenseAlpha=off  SenseQDDot=off  SenseRDDot=off  SenseX=on  SenseY=on  SenseZ=on  SenseXYZ=off  SenseRad=off  SenseAzim=off  SenseDist=off  SenseInc=off  SenseXDot=off  SenseYDot=off  SenseZDot=off  SenseXYZDot=off  SenseRadDot=off  SenseAzimDot=off  SenseDistDot=off  SenseIncDot=off  SenseXDDot=off  SenseYDDot=off  SenseZDDot=off  SenseXYZDDot=off  SenseRadDDot=off  SenseAzimDDot=off  SenseDistDDot=off  SenseIncDDot=off
  to Homogeneous transform{1..6} (6 alike) : robotcorelib/Coordinate Transformation Conversion  InputRepresentation=Rotation Matrix  InputEulerSequence=ZYX  ShowTrVecInputPort=on  OutputRepresentation=Homogeneous Transformation  OutputEulerSequence=ZYX  ShowTrVecOutputPort=on  SimulateUsing=Code generation
  Conn1 : PMIOPort  Side=Right
  g_I0 : Outport
  q_m : Outport  Port=2
  q_dot_m : Outport  Port=3
  p1 : Outport  Port=4
  p1_dot : Outport  Port=5
  tag scope: V_I0=global, g_n0=global, g_ni=global, p_n0=global, p_ni=global
  wires:
  Demux2/1 -> Simulink-PS Converter5/1
  Demux2/3 -> Simulink-PS Converter7/1
  PS-Simulink Converter15/1 -> Mux5/6  "q_dot_1 to 3"
  PS-Simulink Converter10/1 -> Mux5/3  "q_dot_1 to 3"
  PS-Simulink Converter25/1 -> to Homogeneous transform1/1
  Gain/1 -> Scope1/1, Demux2/1
  PS-Simulink Converter8/1 -> Mux3/3
  Mux3/1 -> Scope/1, to Homogeneous transform1/2
  PS-Simulink Converter12/1 -> Mux5/2  "q_dot_1 to 3"
  to Homogeneous transform1/1 -> g_I0/1
  PS-Simulink Converter13/1 -> Mux5/4  "q_dot_1 to 3"
  PS-Simulink Converter26/1 -> Mux3/1
  Demux2/7 -> Simulink-PS Converter11/1
  PS-Simulink Converter14/1 -> Mux5/5  "q_dot_1 to 3"
  Demux2/4 -> Simulink-PS Converter8/1
  PS-Simulink Converter11/1 -> Mux5/1  "q_dot_1 to 3"
  PS-Simulink Converter5/1 -> Mux3/2
  Demux2/6 -> Simulink-PS Converter10/1
  Demux2/2 -> Simulink-PS Converter6/1  "f_elbow"
  Demux2/5 -> Simulink-PS Converter9/1
  PS-Simulink Converter27/1 -> Mux6/3  "q_dot_1 to 3"
  PS-Simulink Converter1/1 -> Mux4/1  "q_dot_1 to 3"
  PS-Simulink Converter6/1 -> Mux4/5  "q_dot_1 to 3"
  PS-Simulink Converter30/1 -> Mux6/6  "q_dot_1 to 3"
  PS-Simulink Converter3/1 -> Mux4/3  "q_dot_1 to 3"
  PS-Simulink Converter18/1 -> Mux1/2  "q_dot_1 to 3"
  PS-Simulink Converter31/1 -> Mux6/7  "q_dot_1 to 3"
  PS-Simulink Converter9/1 -> Mux6/2  "q_dot_1 to 3"
  PS-Simulink Converter7/1 -> Mux4/6  "q_dot_1 to 3"
  PS-Simulink Converter2/1 -> Mux4/2  "q_dot_1 to 3"
  PS-Simulink Converter4/1 -> Mux4/4  "q_dot_1 to 3"
  PS-Simulink Converter21/1 -> Mux1/5  "q_dot_1 to 3"
  PS-Simulink Converter23/1 -> Mux1/7  "q_dot_1 to 3"
  PS-Simulink Converter16/1 -> Mux4/7  "q_dot_1 to 3"
  PS-Simulink Converter28/1 -> Mux6/4  "q_dot_1 to 3"
  Mux4/1 -> q_m/1
  Mux1/1 -> q_dot_m/1
  PS-Simulink Converter24/1 -> Mux6/1  "q_dot_1 to 3"
  Mux6/1 -> Terminator1/1
  PS-Simulink Converter20/1 -> Mux1/4  "q_dot_1 to 3"
  PS-Simulink Converter29/1 -> Mux6/5  "q_dot_1 to 3"
  PS-Simulink Converter22/1 -> Mux1/6  "q_dot_1 to 3"
  PS-Simulink Converter17/1 -> Mux1/1  "q_dot_1 to 3"
  PS-Simulink Converter19/1 -> Mux1/3  "q_dot_1 to 3"
  Mux5/1 -> [V_I0], Scope2/1
  Mux2/1 -> to Homogeneous transform6/2, [p_n0]
  PS-Simulink Converter39/1 -> Mux2/1
  PS-Simulink Converter40/1 -> Mux2/2
  PS-Simulink Converter41/1 -> Mux2/3
  PS-Simulink Converter36/1 -> Mux8/2
  PS-Simulink Converter35/1 -> Mux8/1
  PS-Simulink Converter37/1 -> Mux8/3
  PS-Simulink Converter42/1 -> Mux9/2
  PS-Simulink Converter38/1 -> Mux9/1
  PS-Simulink Converter43/1 -> Mux9/3
  PS-Simulink Converter45/1 -> Mux10/2
  PS-Simulink Converter44/1 -> Mux10/1
  PS-Simulink Converter46/1 -> Mux10/3
  Mux11/1 -> to Homogeneous transform2/2, collect positions/1(p_n2)
  PS-Simulink Converter48/1 -> Mux11/2
  PS-Simulink Converter47/1 -> Mux11/1
  PS-Simulink Converter49/1 -> Mux11/3
  collect positions/1(p_ni) -> [p_ni]
  PS-Simulink Converter32/1 -> to Homogeneous transform2/1
  PS-Simulink Converter33/1 -> to Homogeneous transform3/1
  Mux10/1 -> to Homogeneous transform3/2, collect positions/2(p_n3)
  Mux9/1 -> to Homogeneous transform4/2, collect positions/3(p_n4)
  PS-Simulink Converter34/1 -> to Homogeneous transform4/1
  PS-Simulink Converter50/1 -> to Homogeneous transform5/1
  Mux8/1 -> to Homogeneous transform5/2, collect positions/4(p_n5)
  collect positions1/1(g_ni) -> [g_ni]
  PS-Simulink Converter51/1 -> to Homogeneous transform6/1
  to Homogeneous transform6/1 -> collect positions/5(g_n0), collect positions1/5(g_n0), [g_n0]
  to Homogeneous transform2/1 -> collect positions1/1(g_n2)
  to Homogeneous transform3/1 -> collect positions1/2(g_n3)
  to Homogeneous transform4/1 -> collect positions1/3(g_n4)
  to Homogeneous transform5/1 -> collect positions1/4(g_n5)
  Orbit/1(p1) -> p1/1
  Orbit/2(V_orbit_I) -> p1_dot/1
  fm/1 -> Gain/1
  connections:
  Base Sensing1/LConn1 -- Orbit/RConn1 -- ee_joint/LConn1
  ee_joint/RConn1 -- p_n0/RConn1 -- Base Sensing1/RConn1 -- joint/link7/RConn1
  joint/link4/LConn1 -- p_n4/RConn1 -- joint/link3/RConn1
  Base Sensing1/RConn10 -- PS-Simulink Converter12/LConn1
  Simulink-PS Converter9/RConn1 -- joint/link3/LConn2
  Simulink-PS Converter8/RConn1 -- joint/link4/LConn2
  Base Sensing1/RConn2 -- PS-Simulink Converter25/LConn1
  joint/link5/LConn1 -- joint/link4/RConn1 -- p_n3/RConn1
  Base Sensing1/RConn5 -- PS-Simulink Converter15/LConn1
  Base Sensing1/RConn7 -- PS-Simulink Converter5/LConn1
  joint/link6/LConn1 -- joint/link5/RConn1 -- p_n2/RConn1
  Base Sensing1/RConn11 -- PS-Simulink Converter10/LConn1
  Base Sensing1/RConn3 -- PS-Simulink Converter13/LConn1
  Simulink-PS Converter5/RConn1 -- joint/link7/LConn2
  Base Sensing1/RConn4 -- PS-Simulink Converter14/LConn1
  Base Sensing1/RConn9 -- PS-Simulink Converter11/LConn1
  Base Sensing1/RConn8 -- PS-Simulink Converter8/LConn1
  Base Sensing1/RConn6 -- PS-Simulink Converter26/LConn1
  Simulink-PS Converter7/RConn1 -- joint/link5/LConn2
  joint/link6/RConn3 -- PS-Simulink Converter18/LConn1
  joint/link6/RConn4 -- PS-Simulink Converter9/LConn1
  joint/link5/RConn2 -- PS-Simulink Converter3/LConn1
  joint/link5/RConn3 -- PS-Simulink Converter19/LConn1
  joint/link5/RConn4 -- PS-Simulink Converter27/LConn1
  joint/link4/RConn2 -- PS-Simulink Converter4/LConn1
  joint/link4/RConn3 -- PS-Simulink Converter20/LConn1
  joint/link4/RConn4 -- PS-Simulink Converter28/LConn1
  joint/link3/RConn2 -- PS-Simulink Converter6/LConn1
  joint/link3/RConn3 -- PS-Simulink Converter21/LConn1
  joint/link3/RConn4 -- PS-Simulink Converter29/LConn1
  joint/link6/RConn1 -- joint/link7/LConn1
  joint/link6/RConn2 -- PS-Simulink Converter2/LConn1
  joint/link6/LConn2 -- Simulink-PS Converter6/RConn1
  joint/link7/RConn2 -- PS-Simulink Converter1/LConn1
  joint/link7/RConn3 -- PS-Simulink Converter17/LConn1
  joint/link7/RConn4 -- PS-Simulink Converter24/LConn1
  join/link 1/LConn2 -- Simulink-PS Converter11/RConn1
  join/link 1/LConn1 -- Spacecraft/RConn1
  join/link 1/RConn1 -- joint/link2/LConn1
  Simulink-PS Converter10/RConn1 -- joint/link2/LConn2
  joint/link3/LConn1 -- p_n5/RConn1 -- joint/link2/RConn1
  join/link 1/RConn2 -- PS-Simulink Converter16/LConn1
  PS-Simulink Converter7/LConn1 -- joint/link2/RConn2
  joint/link2/RConn4 -- PS-Simulink Converter30/LConn1
  join/link 1/RConn4 -- PS-Simulink Converter31/LConn1
  joint/link2/RConn3 -- PS-Simulink Converter22/LConn1
  join/link 1/RConn3 -- PS-Simulink Converter23/LConn1
  PS-Simulink Converter41/LConn1 -- p_n0/RConn5
  p_n0/RConn4 -- PS-Simulink Converter40/LConn1
  Spacecraft/LConn1 -- p_n2/LConn1 -- p_n3/LConn1 -- p_n4/LConn1 -- p_n5/LConn1 -- p_n0/LConn1
  p_n0/RConn3 -- PS-Simulink Converter39/LConn1
  PS-Simulink Converter37/LConn1 -- p_n5/RConn5
  p_n5/RConn3 -- PS-Simulink Converter35/LConn1
  p_n5/RConn4 -- PS-Simulink Converter36/LConn1
  PS-Simulink Converter43/LConn1 -- p_n4/RConn5
  p_n4/RConn3 -- PS-Simulink Converter38/LConn1
  p_n4/RConn4 -- PS-Simulink Converter42/LConn1
  PS-Simulink Converter46/LConn1 -- p_n3/RConn5
  p_n3/RConn3 -- PS-Simulink Converter44/LConn1
  p_n3/RConn4 -- PS-Simulink Converter45/LConn1
  PS-Simulink Converter49/LConn1 -- p_n2/RConn5
  p_n2/RConn3 -- PS-Simulink Converter47/LConn1
  p_n2/RConn4 -- PS-Simulink Converter48/LConn1
  PS-Simulink Converter32/LConn1 -- p_n2/RConn2
  p_n3/RConn2 -- PS-Simulink Converter33/LConn1
  p_n4/RConn2 -- PS-Simulink Converter34/LConn1
  p_n5/RConn2 -- PS-Simulink Converter50/LConn1
  p_n0/RConn2 -- PS-Simulink Converter51/LConn1
  Conn1/RConn1 -- Orbit/RConn2

== system KUKA_EE_Controller_v22_orbital_verification2/Dynamic Parameters/A_connection1 ==
  M0 : Inport
  M0m : Inport  Port=2
  Divide : Product  Inputs=/*  Multiplication=Matrix(*)
  A : Outport
  wires:
  Divide/1 -> A/1
  M0/1 -> Divide/1
  M0m/1 -> Divide/2

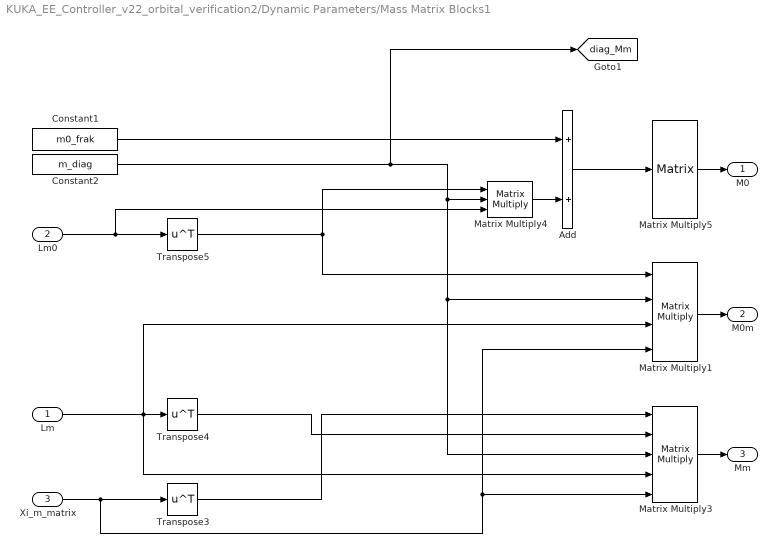
== system KUKA_EE_Controller_v22_orbital_verification2/Dynamic Parameters/Mass Matrix Blocks1 ==
  Lm : Inport
  Lm0 : Inport  Port=2
  Xi_m_matrix : Inport  Port=3
  Add : Sum
  Constant1 : Constant  Value=m0_frak  VectorParams1D=off
  Constant2 : Constant  Value=m_diag  VectorParams1D=off
  Matrix Multiply1 : Product  Inputs=4  Multiplication=Matrix(*)
  Matrix Multiply3 : Product  Inputs=5  Multiplication=Matrix(*)
  Matrix Multiply4 : Product  Inputs=3  Multiplication=Matrix(*)
  Matrix Multiply5 : Product  Inputs=1  Multiplication=Matrix(*)
  Transpose3 : Math  Operator=transpose
  Transpose4 : Math  Operator=transpose
  Transpose5 : Math  Operator=transpose
  M0 : Outport
  M0m : Outport  Port=2
  Mm : Outport  Port=3
  tag scope: diag_Mm=global
  wires:
  Xi_m_matrix/1 -> Matrix Multiply1/4, Matrix Multiply3/5, Transpose3/1
  Matrix Multiply5/1 -> M0/1
  Lm0/1 -> Transpose5/1, Matrix Multiply4/3
  Transpose5/1 -> Matrix Multiply4/1, Matrix Multiply1/1
  Transpose4/1 -> Matrix Multiply3/2
  Matrix Multiply3/1 -> Mm/1
  Matrix Multiply1/1 -> M0m/1
  Matrix Multiply4/1 -> Add/2
  Transpose3/1 -> Matrix Multiply3/1
  Lm/1 -> Matrix Multiply1/3, Matrix Multiply3/4, Transpose4/1
  Add/1 -> Matrix Multiply5/1
  Constant2/1 -> Matrix Multiply4/2, Matrix Multiply3/3, Matrix Multiply1/2, [diag_Mm]
  Constant1/1 -> Add/1
